simulink model "regbot_freja_model"  (R2017b)
settings: Solver=VariableStepAuto  StartTime=0.0  StopTime=1.0  RelTol=1e-3
values from neighbouring files (symbols this model uses):
  Bm = 2e-6    (= 2e-06)    [konstanter.m]    (also in udregninger.m = (Ia*Ktau)/omega)
  G = 9.68    [konstanter.m]    (also in udregninger.m)
  Jm = 5e-6    (= 5e-06)    [konstanter.m]
  Kemf = Ktau    (= 0.02)    [konstanter.m]    (also in udregninger.m = Vemf/omega)
  Ktau = 0.02    [konstanter.m]    (also in udregninger.m = Kemf)
  La = 0.02    [konstanter.m]
  Ra = 4    [konstanter.m]    (also in udregninger.m = (Va-Vemf)/Ia)
  rw = 0.03    [konstanter.m]    (also in udregninger.m)
settings Model: Creator=irene  LastModifiedBy=asger
settings CodeAppCC: StateflowObjectComments=on

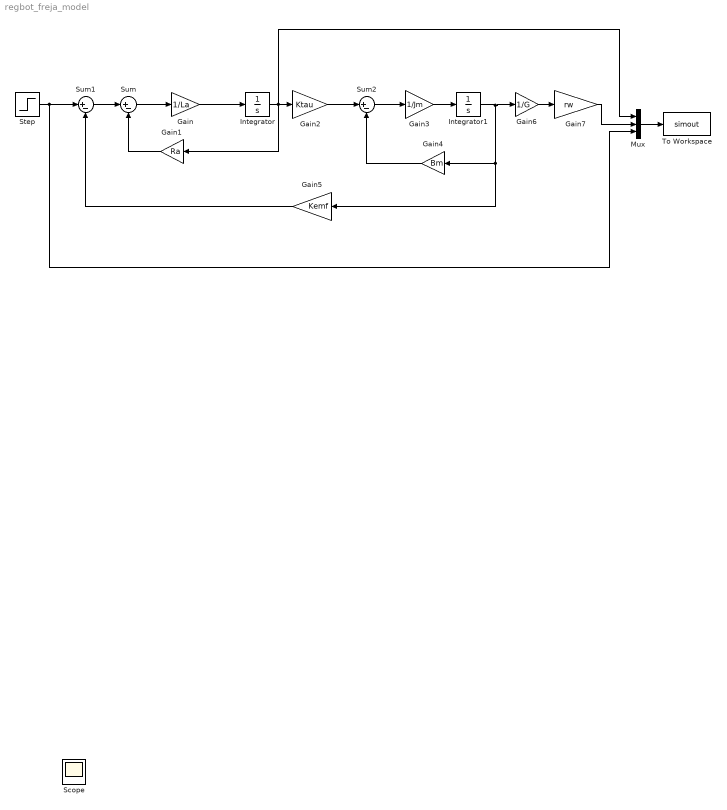
== system regbot_freja_model ==
  Gain : Gain  Gain=1/La
  Gain1 : Gain  Gain=Ra
  Gain2 : Gain  Gain=Ktau
  Gain3 : Gain  Gain=1/Jm
  Gain4 : Gain  Gain=Bm
  Gain5 : Gain  Gain=Kemf
  Gain6 : Gain  Gain=1/G
  Gain7 : Gain  Gain=rw
  Integrator : Integrator
  Integrator1 : Integrator
  Mux : Mux  Inputs=3
  Step : Step  Time=0.5  Before=3  After=4  SampleTime=0
  Sum : Sum  Inputs=|+-
  Sum1 : Sum  Inputs=|+-
  Sum2 : Sum  Inputs=|+-
  To Workspace : ToWorkspace  VariableName=simout  SaveFormat=Timeseries  SampleTime=-1
  Scope : Scope
  wires:
  Gain2/1 -> Sum2/1
  Gain3/1 -> Integrator1/1
  Sum1/1 -> Sum/1
  Sum/1 -> Gain/1
  Sum2/1 -> Gain3/1
  Integrator1/1 -> Gain5/1, Gain4/1, Gain6/1
  Gain4/1 -> Sum2/2
  Gain5/1 -> Sum1/2
  Gain1/1 -> Sum/2
  Step/1 -> Mux/3, Sum1/1
  Gain6/1 -> Gain7/1
  Gain/1 -> Integrator/1
  Integrator/1 -> Mux/1, Gain1/1, Gain2/1
  Gain7/1 -> Mux/2
  Mux/1 -> To Workspace/1
